simulink model "show_image"  (R2021a)
settings: Solver=VariableStepAuto  StartTime=0.0  StopTime=10.0  RelTol=1e-3
libraries: visionsources x1, visionsinks x1
settings Model: Creator=BPRIDDY  LastModifiedBy=BPRIDDY

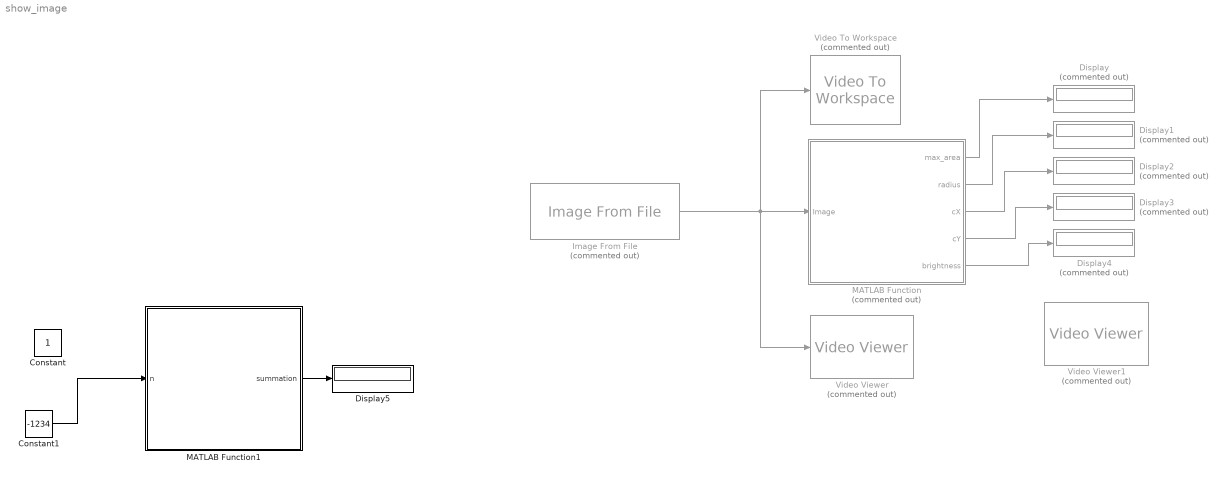
== system show_image ==
  Constant : Constant  VectorParams1D=off
  Constant1 : Constant  Value=-1234  VectorParams1D=off
  Display{,1..4} (5 alike) : Display  Commented=on
  Display5 : Display
  Image From File : visionsources/Image From File  Tag=vipblks_nd  Commented=on  FileName=C:\Users\bpriddy\Documents\GitHub\Senior-Design\save\video_ai\whole916.png  Ts=inf  imagePorts=One multidimensional signal  OutPortLabels=R|G|B  ImageDataType=Inherit from input image  sdImageDataType=uint(8)  Signed=on  WordLength=16  FractionLengthMode=User-defined  FractionLength=15
  MATLAB Function : MATLAB Function  Commented=on  TreatAsAtomicUnit=on
  MATLAB Function1 : MATLAB Function  TreatAsAtomicUnit=on
  Video To Workspace : visionsinks/Video To Workspace  Commented=on  VariableName=vout  NumInputs=1  DataLimit=10  DecimationFactor=1  LogFi=off  InPortLabels=R|G|B
      settings: SourceProductBaseCode=VP
  Video Viewer : VideoViewer  Commented=on  FigPos=[644 646 418 304]
  Video Viewer1 : VideoViewer  Commented=on  FigPos=[2041 741 418 304]
  wires:
  Constant1/1 -> MATLAB Function1/1(n)
  MATLAB Function1/1(summation) -> Display5/1
  MATLAB Function/1(max_area) -> Display/1
  MATLAB Function/2(radius) -> Display1/1
  MATLAB Function/5(brightness) -> Display4/1
  MATLAB Function/4(cY) -> Display3/1
  Image From File/1 -> Video To Workspace/1, MATLAB Function/1(Image), Video Viewer/1
  MATLAB Function/3(cX) -> Display2/1

== matlab function show_image/MATLAB Function1 ==
  data: n input; summation output
function summation  = summmmm(n)
    %py.importlib.import_module('test');
    coder.extrinsic('py.importlib.import_module.test')
    summation = test.Absolute(n)
    
end

== matlab function show_image/MATLAB Function ==
  data: Image input; max_area output; radius output; cX output; cY output; brightness output

% if count(py.sys.path,'') == 0
%     insert(py.sys.path,int32(0),'');
% end
function [max_area, radius, cX, cY, brightness] = process_image(Image)
    
%     if count(py.sys.path,'') == 0
%             insert(py.sys.path,int32(0),'');
%     end
    [max_area, radius, cX, cY, brightness] = py.process_frame_python.process_frame(Image)
    

end
